simulink model "P_PI_PID"  (R2019b)
settings: Solver=FixedStepAuto  StartTime=0.0  StopTime=20.0  FixedStep=1e-3  MinStep=1e-15  RelTol=1e-5
values from neighbouring files (symbols this model uses):
  D3 = P_kr/COEF_D3    (= 1.23333333333)    [code6.m]
  I2 = P_kr/COEF_I2    (= 1.85)    [code6.m]
  I3 = P_kr/COEF_I3    (= 1.85)    [code6.m]
  P1 = COEF_P1*K_kr    [code6.m]
  P2 = COEF_P2*K_kr    [code6.m]
  P3 = COEF_P3*K_kr    [code6.m]
settings Model: Creator=Szymon  LastModifiedBy=Szymon

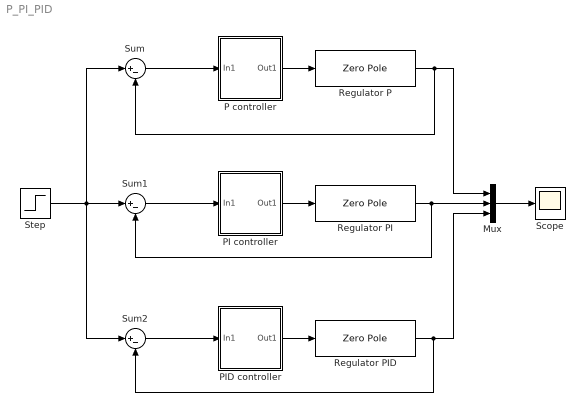
== system P_PI_PID ==
  Mux : Mux  Inputs=3
  P controller : Subsystem  mask{P=P1}
  PI controller : Subsystem  mask{P=P2, I=I2}
  PID controller : Subsystem  mask{P=P3, I=I3, D=D3}
  Regulator P : ZeroPole  Zeros=[]  Poles=[-1 -1 -1]
  Regulator PI : ZeroPole  Zeros=[]  Poles=[-1 -1 -1]
  Regulator PID : ZeroPole  Zeros=[]  Poles=[-1 -1 -1]
  Scope : Scope
  Step : Step  SampleTime=0
  Sum : Sum  Inputs=|+-
  Sum1 : Sum  Inputs=|+-
  Sum2 : Sum  Inputs=|+-
  wires:
  Mux/1 -> Scope/1
  Regulator PI/1 -> Sum1/2, Mux/2
  Regulator P/1 -> Sum/2, Mux/1
  Regulator PID/1 -> Sum2/2, Mux/3
  PI controller/1(Out1) -> Regulator PI/1
  Sum1/1 -> PI controller/1(In1)
  Sum2/1 -> PID controller/1(In1)
  PID controller/1(Out1) -> Regulator PID/1
  P controller/1(Out1) -> Regulator P/1
  Sum/1 -> P controller/1(In1)
  Step/1 -> Sum2/1, Sum/1, Sum1/1

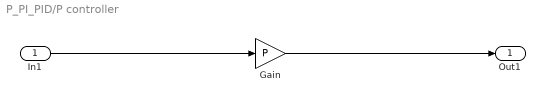
== system P_PI_PID/P controller ==
  In1 : Inport
  Gain : Gain  Gain=P
  Out1 : Outport
  wires:
  Gain/1 -> Out1/1
  In1/1 -> Gain/1

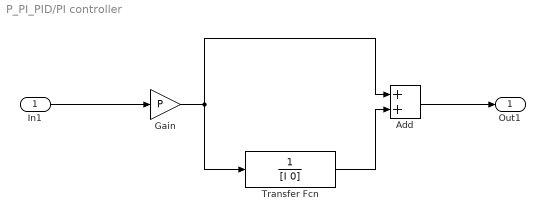
== system P_PI_PID/PI controller ==
  In1 : Inport
  Add : Sum
  Gain : Gain  Gain=P
  Transfer Fcn : TransferFcn  Denominator=[I 0]
  Out1 : Outport
  wires:
  Gain/1 -> Add/1, Transfer Fcn/1
  Add/1 -> Out1/1
  Transfer Fcn/1 -> Add/2
  In1/1 -> Gain/1

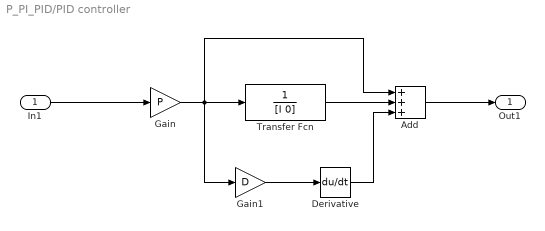
== system P_PI_PID/PID controller ==
  In1 : Inport
  Add : Sum  Inputs=+++
  Derivative : Derivative
  Gain : Gain  Gain=P
  Gain1 : Gain  Gain=D
  Transfer Fcn : TransferFcn  Denominator=[I 0]
  Out1 : Outport
  wires:
  Gain1/1 -> Derivative/1
  Derivative/1 -> Add/3
  Gain/1 -> Add/1, Gain1/1, Transfer Fcn/1
  Add/1 -> Out1/1
  Transfer Fcn/1 -> Add/2
  In1/1 -> Gain/1
